simulink model "Q5OndaCompletaRControlavel"  (R2016a)
settings: Solver=VariableStepAuto  StartTime=0.0  StopTime=1/60  RelTol=1e-3
undefined symbols (not defined in the file or in its folder): alpha
libraries: powerlib x16
settings Model: Creator=MATHEUS  LastModifiedBy=MATHEUS
settings SimscapeCC: SimscapeLogType=all  SimscapeLogOpenViewer=on

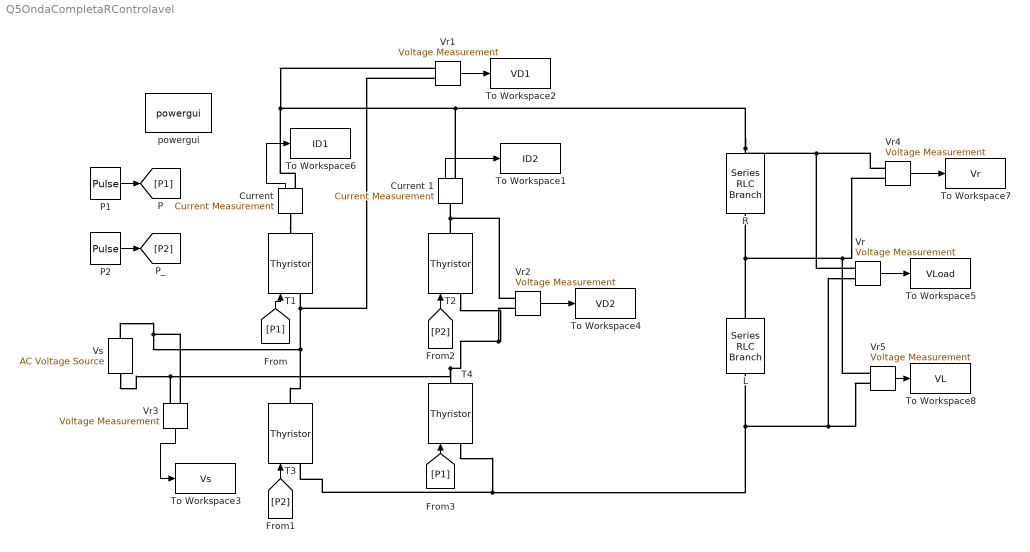
== system Q5OndaCompletaRControlavel ==
  "Current " : powerlib/Measurements/Current Measurement  PhasorSimulation=off  OutputType=Complex  PSBequivalent=0
  Current 1 : powerlib/Measurements/Current Measurement  PhasorSimulation=off  OutputType=Complex  PSBequivalent=0
  L : powerlib/Elements/Series RLC Branch  LConnTagsString=__new0  RConnTagsString=__new0  BranchType=L  Resistance=100  Inductance=1  SetiL0=off  InitialCurrent=0  Capacitance=1e-6  Setx0=off  InitialVoltage=0  Measurements=None
  P1 : DiscretePulseGenerator  PulseType=Time based  Period=1/60  PulseWidth=10  PhaseDelay=(alpha)/(2*pi*60)
  P2 : DiscretePulseGenerator  PulseType=Time based  Period=1/60  PulseWidth=10  PhaseDelay=(alpha + pi)/(2*pi*60)
  R : powerlib/Elements/Series RLC Branch  LConnTagsString=__new0  RConnTagsString=__new0  BranchType=R  Resistance=100  Inductance=0.1  SetiL0=off  InitialCurrent=0  Capacitance=1e-6  Setx0=off  InitialVoltage=0  Measurements=None
  T{1..4} (4 alike) : powerlib/Power Electronics/Thyristor  Ron=0.001  Lon=0  Vf=0  IC=0  Rs=500  Cs=250e-9  Measurements=off
  To Workspace1 : ToWorkspace  VariableName=ID2  SaveFormat=Structure With Time  SampleTime=-1
      settings: Save2DSignal=2-D array (concatenate along first dimension)
  To Workspace2 : ToWorkspace  VariableName=VD1  SaveFormat=Structure With Time  SampleTime=-1
      settings: Save2DSignal=2-D array (concatenate along first dimension)
  To Workspace3 : ToWorkspace  VariableName=Vs  SaveFormat=Structure With Time  SampleTime=-1
  To Workspace4 : ToWorkspace  VariableName=VD2  SaveFormat=Structure With Time  SampleTime=-1
      settings: Save2DSignal=2-D array (concatenate along first dimension)
  To Workspace5 : ToWorkspace  VariableName=VLoad  SaveFormat=Structure With Time  SampleTime=-1
      settings: Save2DSignal=2-D array (concatenate along first dimension)
  To Workspace6 : ToWorkspace  VariableName=ID1  SaveFormat=Structure With Time  SampleTime=-1
      settings: Save2DSignal=2-D array (concatenate along first dimension)
  To Workspace7 : ToWorkspace  VariableName=Vr  SaveFormat=Structure With Time  SampleTime=-1
      settings: Save2DSignal=2-D array (concatenate along first dimension)
  To Workspace8 : ToWorkspace  VariableName=VL  SaveFormat=Structure With Time  SampleTime=-1
      settings: Save2DSignal=2-D array (concatenate along first dimension)
  Vr{,1..5} (6 alike) : powerlib/Measurements/Voltage Measurement  PhasorSimulation=off  OutputType=Complex  PSBequivalent=0
  Vs : powerlib/Electrical Sources/AC Voltage Source  Amplitude=100*sqrt(2)  Phase=0  Frequency=60  SampleTime=0  Measurements=Voltage  BusType=swing  Pref=10e3  Qref=0  Qmin=-inf  Qmax=+inf
  powergui : powerlib/powergui  Priority=1  SimulationMode=Continuous  SolverType=Tustin/Backward Euler (TBE)  SampleTime=50e-6  frequency=60  SPID=off  DisableSnubberDevices=off  DisableRonSwitches=off  DisableVfSwitches=off  SwTol=0  DisplayEquations=off  Interpol=off  ExternalGateDelay=off  methode=off  Ts=10  FunctionMessages=off  echomessages=off  HookPort=off  EnableUseOfTLC=off  x0status=blocks  frequencyindice=60  Pbase=100e6  ErrMax=1e-4  Iterations=50  UnitsV=kV  UnitsW=MW  buscounter=0  RestoreLinks=warning  ResistiveCurrentMeasurement=off  Frange=[0:2:500]  Ylog=off  Xlog=on  ShowGrid=off  save=off  variable=ZData  structure=VR  ZoomFFT=off  StartTime=0.0  cycles=1  DisplayStyle=1  fundamental=60  FreqAxis=off  MaxFrequency=1000  frequencyindicesteady=1  RmsSteady=1  display=off
  wires:
  Vr/1 -> To Workspace5/1
  P1/1 -> [P1]
  [P1] -> T1/1
  [P2] -> T3/1
  [P2] -> T2/1
  [P1] -> T4/1
  Vr1/1 -> To Workspace2/1
  P2/1 -> [P2]
  Vr2/1 -> To Workspace4/1
  Vr3/1 -> To Workspace3/1
  Current 1/1 -> To Workspace1/1
  "Current "/1 -> To Workspace6/1
  Vr4/1 -> To Workspace7/1
  Vr5/1 -> To Workspace8/1
  connections:
  Vr1/LConn1 -- Vr/LConn1 -- Vr4/LConn1 -- R/RConn1 -- Current 1/RConn1 -- "Current "/RConn1
  T4/LConn1 -- Vr5/LConn2 -- Vr/LConn2 -- L/LConn1 -- T3/LConn1
  T2/LConn1 -- Vr2/LConn2 -- Vs/LConn1 -- Vr3/LConn2 -- T4/RConn1
  T3/RConn1 -- Vr3/LConn1 -- Vs/RConn1 -- Vr1/LConn2 -- T1/LConn1
  "Current "/LConn1 -- T1/RConn1
  T2/RConn1 -- Vr2/LConn1 -- Current 1/LConn1
  L/RConn1 -- Vr5/LConn1 -- Vr4/LConn2 -- R/LConn1
